simulink model "Lab2_first_graph"  (R2024a)
settings: Solver=VariableStepAuto  StartTime=0.0  StopTime=10.0  RelTol=1e-3
libraries: commchan3 x1, dspfdesign x1, dspmlti4 x1
settings Model: Creator=pyrpo  LastModifiedBy=pyrpo

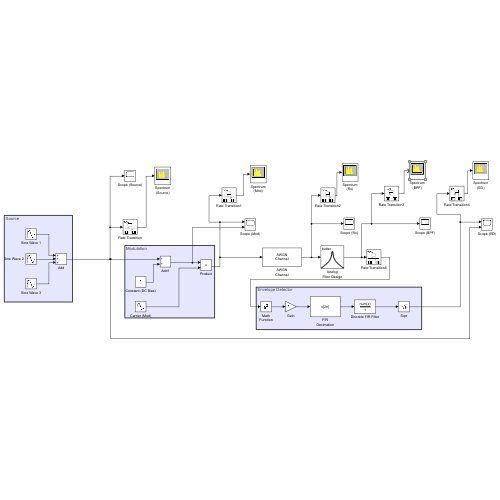
[thumbnail: Simulink's stored preview of the top-level diagram]
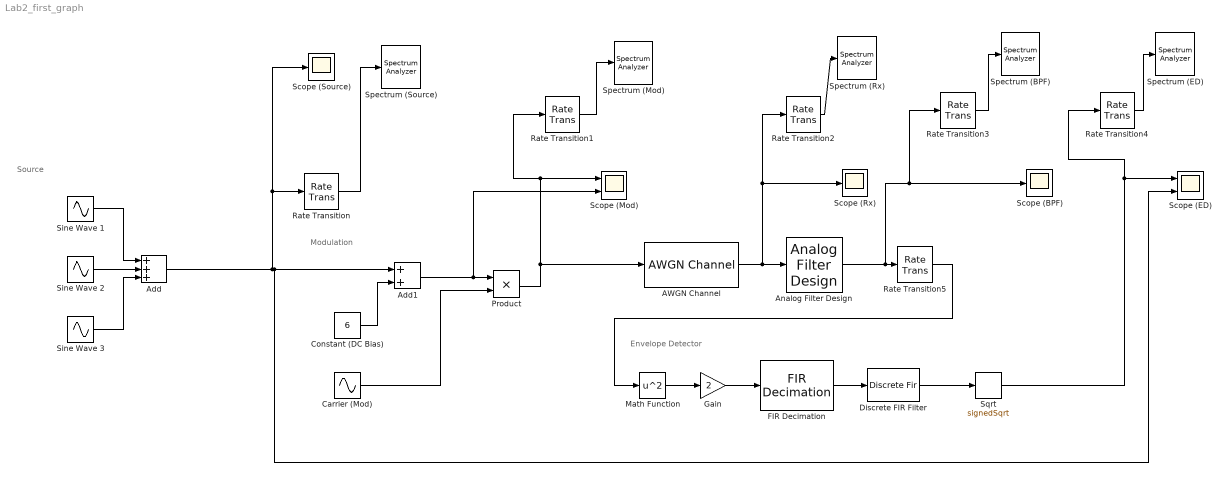
== system Lab2_first_graph ==
  note: Envelope Detector
  note: Modulation
  note: Source
  AWGN Channel : commchan3/AWGN Channel  LegacyMode=off  NoiseMethod=Variance  noiseMode="Signal to noise ratio  (SNR)"  EbNo=10  EsNo=10  SNR=10  BitsPerSymbol=1  SignalPower=1  SamplesPerSymbol=1  SymbolPeriod=1  VarianceSource=Parameter  Variance=1e-2  RandomStream=Global stream  Seed=67  SimulateUsing=Code generation
  Add : Sum  Inputs=+++
  Add1 : Sum
  Analog Filter Design : dspfdesign/Analog Filter Design  method=Butterworth  filttype=Bandpass  N=8  Wlo=14300*2*pi  Whi=15800*2*pi  Rp=2  Rs=40
  Carrier (Mod) : Sin  Frequency=30000*pi  Phase=pi/2  SampleTime=0
  Constant (DC Bias) : Constant  Value=6
  Discrete FIR Filter : DiscreteFir  Coefficients=firpm(20,[0 0.03 0.1 1], [1 1 0 0])
  FIR Decimation : dspmlti4/FIR Decimation  FilterSource=Dialog parameters  h=[1 1]  D=2  filtStruct=Direct form  FilterObject=FDECIM  framing=Enforce single-rate processing  AllowArbitraryInputLength=off  inputOffset=0  outputBufInitCond=0  roundingMode=Floor  overflowMode=off  firstCoeffDataTypeStr=Inherit: Same word length as input  firstCoeffMin=[]  firstCoeffMax=[]  firstCoeffLastDataTypeStr=Inherit: Same word length as input  outputDataTypeStr=Inherit: Same as accumulator  outputMin=[]  outputMax=[]  outputLastDataTypeStr=Inherit: Same as accumulator
  Gain : Gain  Gain=2
  Math Function : Math  Operator=square
  Product : Product
  Rate Transition{,1..5} (6 alike) : RateTransition  OutPortSampleTime=2e-5
  Scope (BPF) : Scope
  Scope (ED) : Scope  NumInputPorts=2
  Scope (Mod) : Scope  NumInputPorts=2
  Scope (Rx) : Scope
  Scope (Source) : Scope
  Sine Wave 1 : Sin  Frequency=1000*pi  SampleTime=0
  Sine Wave 2 : Sin  Amplitude=3  Frequency=600*pi  SampleTime=0
  Sine Wave 3 : Sin  Amplitude=1.5  Frequency=1200*pi  SampleTime=0
  Spectrum (BPF) : SpectrumAnalyzer  WindowPosition=[0.000000,36.000000,1536.000000,792.000000,]  ScopeFrameLocation=window  YLimits=[-38.68673621,48.15422087]  SelectedToolstripTab=spectrumAnalyzerToolstrip.measurementsTab
  Spectrum (ED) : SpectrumAnalyzer  WindowPosition=[0.000000,36.000000,1536.000000,792.000000,]  ScopeFrameLocation=window  RBW=1  YLimits=[-120.1629039,67.75974112]  SelectedToolstripTab=spectrumAnalyzerToolstrip.estimationTab
  Spectrum (Mod) : SpectrumAnalyzer  WindowPosition=[0.000000,36.000000,1536.000000,792.000000,]  ScopeFrameLocation=window  YLimits=[-27.97115231,46.40132462]  SelectedToolstripTab=spectrumAnalyzerToolstrip.channelMeasurementsTab
  Spectrum (Rx) : SpectrumAnalyzer  WindowPosition=[0.000000,36.000000,1536.000000,792.000000,]  ScopeFrameLocation=window  YLimits=[-29.40234738,46.56202468]  SelectedToolstripTab=spectrumAnalyzerToolstrip.measurementsTab
  Spectrum (Source) : SpectrumAnalyzer  WindowPosition=[0.000000,36.000000,1536.000000,792.000000,]  ScopeFrameLocation=window  YLimits=[-34.50902388,40.71788721]  SelectedToolstripTab=spectrumAnalyzerToolstrip.channelMeasurementsTab
  Sqrt : Sqrt  Operator=signedSqrt
  wires:
  Sine Wave 1/1 -> Add/1
  Sine Wave 2/1 -> Add/2
  Sine Wave 3/1 -> Add/3
  AWGN Channel/1 -> Analog Filter Design/1, Rate Transition2/1, Scope (Rx)/1
  Add/1 -> Add1/1, Scope (ED)/2, Scope (Source)/1, Rate Transition/1
  Constant (DC Bias)/1 -> Add1/2
  Add1/1 -> Product/1, Scope (Mod)/2
  Carrier (Mod)/1 -> Product/2
  Product/1 -> AWGN Channel/1, Rate Transition1/1, Scope (Mod)/1
  Analog Filter Design/1 -> Scope (BPF)/1, Rate Transition3/1, Rate Transition5/1
  Math Function/1 -> Gain/1
  Gain/1 -> FIR Decimation/1
  FIR Decimation/1 -> Discrete FIR Filter/1
  Discrete FIR Filter/1 -> Sqrt/1
  Rate Transition5/1 -> Math Function/1
  Sqrt/1 -> Rate Transition4/1, Scope (ED)/1
  Rate Transition4/1 -> Spectrum (ED)/1
  Rate Transition/1 -> Spectrum (Source)/1
  Rate Transition1/1 -> Spectrum (Mod)/1
  Rate Transition2/1 -> Spectrum (Rx)/1
  Rate Transition3/1 -> Spectrum (BPF)/1
